simulink model "CollectMechanism"  (R2019b)
settings: Solver=VariableStepAuto  StartTime=0.0  StopTime=0.8  RelTol=1e-3
values from neighbouring files (symbols this model uses):
  GR = 1/27    (= 0.037037037037)    [ParamMechanism.m]
  J = 15.7/100/100/1000    (= 1.57e-06)    [ParamMotor.m]
  Kb = Kt    (= 0.0029)    [ParamMotor.m]
  Kd = 0    [ParamPID.m]
  Kf = 0    [ParamMotor.m]
  Ki = 0    [ParamPID.m]
  Kp = 1.3    [ParamPID.m]
  Kt = 2.9E-3    (= 0.0029)    [ParamMotor.m]
  L = 0.034E-3    (= 3.4e-05)    [ParamMotor.m]
  R = 0.196    [ParamMotor.m]
  RadToPos = 0.122/(2*pi)    (= 0.0194169030572)    [ParamMechanism.m]
  RaitoToV = 12.0    (= 12)    [ParamMechanism.m]
  targetPos = 0.25    [ParamMechanism.m]
  Td = 0    [ParamMechanism.m]
settings Model: Creator=ryoga  LastModifiedBy=ryoga

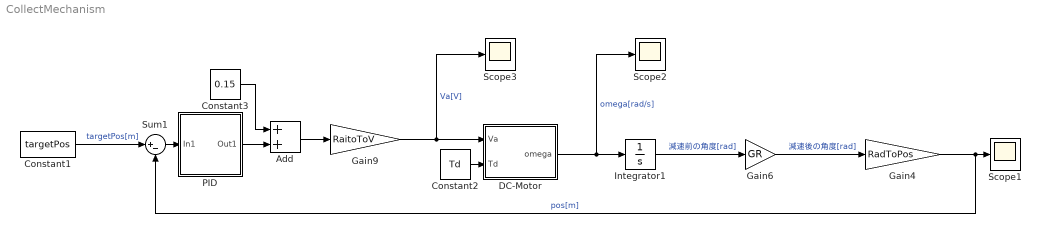
== system CollectMechanism ==
  Add : Sum
  Constant1 : Constant  Value=targetPos
  Constant2 : Constant  Value=Td
  Constant3 : Constant  Value=0.15
  DC-Motor : Subsystem
  Gain4 : Gain  Gain=RadToPos
  Gain6 : Gain  Gain=GR
  Gain9 : Gain  Gain=RaitoToV
  Integrator1 : Integrator
  PID : Subsystem
  Scope1 : Scope
  Scope2 : Scope
  Scope3 : Scope
  Sum1 : Sum  Inputs=|+-
  wires:
  Integrator1/1 -> Gain6/1  "減速前の角度[rad]"
  DC-Motor/1(omega) -> Scope2/1, Integrator1/1  "omega[rad/s]"
  Gain6/1 -> Gain4/1  "減速後の角度[rad]"
  Gain4/1 -> Sum1/2, Scope1/1  "pos[m]"
  Constant2/1 -> DC-Motor/2(Td)
  Constant1/1 -> Sum1/1  "targetPos[m]"
  Gain9/1 -> Scope3/1, DC-Motor/1(Va)  "Va[V]"
  Sum1/1 -> PID/1(In1)
  PID/1(Out1) -> Add/2
  Add/1 -> Gain9/1
  Constant3/1 -> Add/1

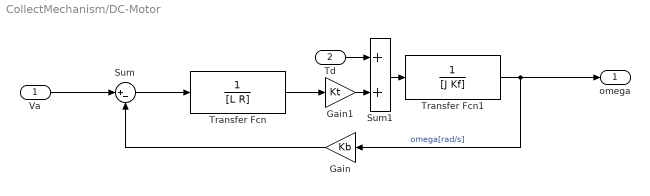
== system CollectMechanism/DC-Motor ==
  Va : Inport
  Td : Inport  Port=2
  Gain : Gain  Gain=Kb
  Gain1 : Gain  Gain=Kt
  Sum : Sum  Inputs=|+-
  Sum1 : Sum
  Transfer Fcn : TransferFcn  Denominator=[L R]
  Transfer Fcn1 : TransferFcn  Denominator=[J Kf]
  omega : Outport
  wires:
  Gain/1 -> Sum/2
  Sum/1 -> Transfer Fcn/1
  Va/1 -> Sum/1
  Transfer Fcn/1 -> Gain1/1
  Transfer Fcn1/1 -> Gain/1, omega/1  "omega[rad/s]"
  Gain1/1 -> Sum1/2
  Sum1/1 -> Transfer Fcn1/1
  Td/1 -> Sum1/1

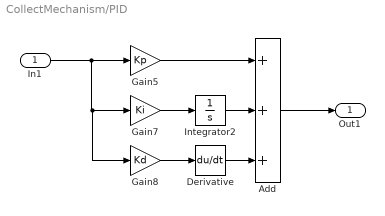
== system CollectMechanism/PID ==
  In1 : Inport
  Add : Sum  Inputs=+++
  Derivative : Derivative
  Gain5 : Gain  Gain=Kp
  Gain7 : Gain  Gain=Ki
  Gain8 : Gain  Gain=Kd
  Integrator2 : Integrator
  Out1 : Outport
  wires:
  Integrator2/1 -> Add/2
  In1/1 -> Gain8/1, Gain7/1, Gain5/1
  Gain5/1 -> Add/1
  Gain7/1 -> Integrator2/1
  Derivative/1 -> Add/3
  Add/1 -> Out1/1
  Gain8/1 -> Derivative/1
